simulink model "Stateflow_graphicFunction"  (R2023b)
settings: Solver=VariableStepAuto  StartTime=0.0  StopTime=10.0  RelTol=1e-3
settings Model: Creator=Administrator  LastModifiedBy=Administrator

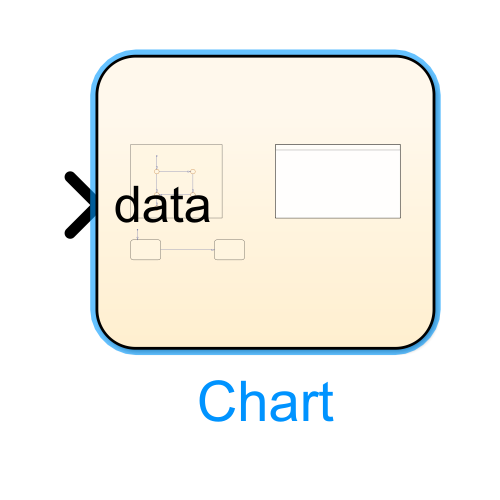
[thumbnail: Simulink's stored preview of the top-level diagram]
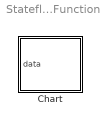
== system Stateflow_graphicFunction ==
  Chart : Stateflow chart  TreatAsAtomicUnit=on

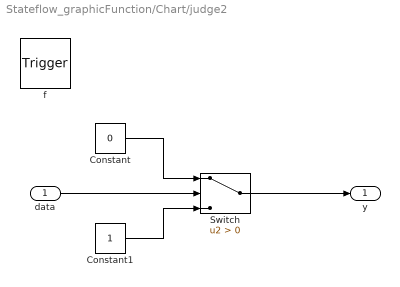
== system Stateflow_graphicFunction/Chart/judge2 ==
  data : Inport  OutDataTypeStr=double  PortDimensions=1
  f : TriggerPort  TriggerType=function-call  VariantControl=(inherit)
      settings: CopyFcn=Stateflow.SLINSF.SimulinkMan.removeBlockPreDeleteFcn  PreDeleteFcn=Stateflow.SLINSF.SimulinkMan.unsafePredeleteFcn
  Constant : Constant  Value=0  OutDataTypeStr=boolean
  Constant1 : Constant  OutDataTypeStr=boolean
  Switch : Switch  Criteria=u2 > Threshold  SaturateOnIntegerOverflow=off  InputSameDT=off
  y : Outport
  wires:
  data/1 -> Switch/2
  Switch/1 -> y/1
  Constant/1 -> Switch/1
  Constant1/1 -> Switch/3

== stateflow chart Stateflow_graphicFunction/Chart ==
  state y = judge [function]
    (default) -> (junction 14) : % a sample demo
    (junction 14) -> (junction 15) [order 1] : [data > 1]
    (junction 14) -> (junction 16) [order 2] : {y = false;}
    (junction 15) -> (junction 17) : {y = true;}
    (junction 17) -> (junction 16)
    (junction 16) -> (junction 18)
  state y = judge2(data) [function]
  state A
  state B
  (default) -> A
  A -> B : [judge2(data)]
  data: y function_output; data function_input double size=1; y function_output; data input
